simulink model "Lab1"  (R2013b)
settings: Solver=ode1  StartTime=0.0  StopTime=1  FixedStep=0.002  RelTol=1e-3
settings Model: ExtModeTrigDuration=5000  Creator=ee128-aai  LastModifiedBy=ee128-aai
settings SolverCC: PositivePriorityOrder=on
settings RTWCC: SystemTargetFile=quarc_win64.tlc  TemplateMakefile=quarc_default_tmf  Description=QUARC Win64 Target  ProcessScript=quarc_win64_make_rtw_hook
settings STFCustomTargetCC: TargetPreCompLibLocation=C:\PROGRA~3\QUARC\lib\2013b\win64\release  GeneratePreprocessorConditionals=Disable all  CombineOutputUpdateFcns=on  GRTInterface=off  SystemTargetFile=quarc_win64.tlc
settings GRTTargetCC: TargetPreCompLibLocation=C:\PROGRA~3\QUARC\lib\2013b\win64\release  ParMdlRefBuildCompliant=off  CompOptLevelCompliant=off  ConcurrentExecutionCompliant=off  MatFileLogging=off  ExtMode=on  ExtModeMexFile=quarc_comm

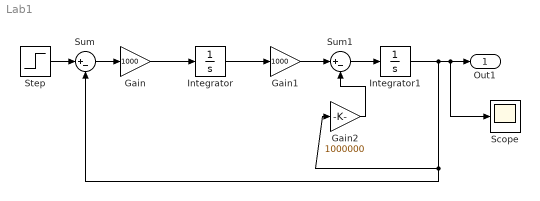
== system Lab1 ==
  Gain : Gain  Gain=1000
  Gain1 : Gain  Gain=1000
  Gain2 : Gain  Gain=1000000
  Integrator : Integrator
  Integrator1 : Integrator
  Scope : Scope
  Step : Step  SampleTime=0
  Sum : Sum  Inputs=|+-
  Sum1 : Sum  Inputs=|+-
  Out1 : Outport
  wires:
  Step/1 -> Sum/1
  Sum/1 -> Gain/1
  Gain/1 -> Integrator/1
  Integrator/1 -> Gain1/1
  Gain1/1 -> Sum1/1
  Sum1/1 -> Integrator1/1
  Integrator1/1 -> Gain2/1, Sum/2, Scope/1, Out1/1
  Gain2/1 -> Sum1/2
